simulink library "mach_lib"  (Simulink 6.3)
undefined symbols (not defined in the file): accel_cmd, aero_surf_qbar_off, aero_surf_qbar_on, altitude_stop, angular_rate_stop, att_cmd_select, att_trim_IC, att_type, att_type_numbers, bb_ellipsoid, bb_params, chi_trim_IC, command_time, compute_all_rate_cols, compute_all_vel_cols, constants, cosA, da_trim_IC, de_trim_IC, DiscIntNeverNeededParam, dr_trim_IC, dtsim, E_rwy, E_trim_IC, Ed_cmd, Ed_trim_IC, energy_stop, eow_boundary, full_surf_llim, full_surf_ulim, gain_var_struct, gam_cmd_descent, gam_cmd_preflare, gamdot_cmd_descent, gamdot_cmd_flare, gamdot_cmd_preflare, gamma_trim_IC, h_trim_IC, hd_cmd, hd_trim_IC, ideal_vel_Kb, integrate_start_time_sim, integrate_state_sim, llim, MACH, MACH_att_fb, MACH_gain_mat, MACH_mass_IC, MACH_pos_IC, MACH_pqr_Bmat_IC, MACH_pqr_IC, MACH_pqr_u_IC, MACH_quat_IC, MACH_throttle_IC, MACH_U_nom_IC, MACH_vel_Bmat_IC, MACH_vel_cvdnom_IC, MACH_vel_IC, MACH_vel_uold_IC, max_chi_cmd ... (+67)
libraries: simulink x75, mach_lib x27, utility_lib x25, model_lib x7, models x6
(part 2 of 6)

== system mach_lib/claw_main/pos_loops ==
  signal_bus : Inport
  outer_cmd : Inport  Port=2
  inner_cmd : Inport  Port=3
  Bus Creator : BusCreator  Inputs=5
  Bus Selector : BusSelector  OutputSignals=feed_forward.pos_ff,mode_sw.int_reset_sw,control_params.pos_desdyn,y_meas.dc_fltpath
  Bus Selector1 : BusSelector  OutputSignals=x_est.NEh
  Mux : Mux  Inputs=[3 1 ]
  P+I+AW+TRIM Control : mach_lib/P+I+AW+TRIM Control
  Product : Product  Multiplication=Matrix(*)  RndMeth=Zero
  Selector1 : Selector  Elements=[1 2 4]  InputPortWidth=4
  Selector3 : Selector  Elements=[1 2 4 3]  InputPortWidth=4
  compute trim : Subsystem
  limiter : Subsystem
  select pos cmd : Subsystem
  d_cmd : Outport
  outputs : Outport  Port=2
  cmd : Outport  Port=3
  wires:
  select pos cmd/2(cam_cmd) -> [camcmd]
  Bus Selector/1 -> P+I+AW+TRIM Control/3  "<pos_ff>"
  limiter/2(cvd_extra) -> [cvdex], Bus Creator/1  "cvdex"
  Product/1 -> Bus Creator/5  "cvdex_fltpath"
  Bus Selector/4 -> Product/1  "<dc_fltpath>"
  Bus Creator/1 -> outputs/1
  P+I+AW+TRIM Control/2 -> Bus Creator/2  "integ"
  [cvdex] -> Product/2
  P+I+AW+TRIM Control/1 -> limiter/3(cvd_des_in)
  limiter/1(cvd_des) -> compute trim/2(cmd), Mux/1
  Bus Selector/3 -> P+I+AW+TRIM Control/7  "<pos_desdyn>"
  Bus Selector/2 -> P+I+AW+TRIM Control/6  "<int_reset_sw>"
  [cvdex] -> P+I+AW+TRIM Control/4
  [trim] -> P+I+AW+TRIM Control/5
  [cv] -> Bus Creator/4  "cv"
  [cvc] -> Bus Creator/3  "cvc"
  Selector3/1 -> d_cmd/1
  select pos cmd/3(cmd) -> cmd/1
  outer_cmd/1 -> select pos cmd/2(outer cmd)
  Selector1/1 -> limiter/1(vel_inner_cmd), compute trim/1(inner cmd)
  inner_cmd/1 -> Selector1/1
  compute trim/1(trim) -> [trim]
  signal_bus/1 -> limiter/2(signal_bus), Bus Selector1/1, select pos cmd/3(signal_bus), Bus Selector/1
  Bus Selector1/1 -> select pos cmd/1(NEh_current), [cv], P+I+AW+TRIM Control/1  "<NEh>"
  select pos cmd/1(NEh_cmd) -> [cvc], P+I+AW+TRIM Control/2
  Mux/1 -> Selector3/1
  [camcmd] -> Mux/2

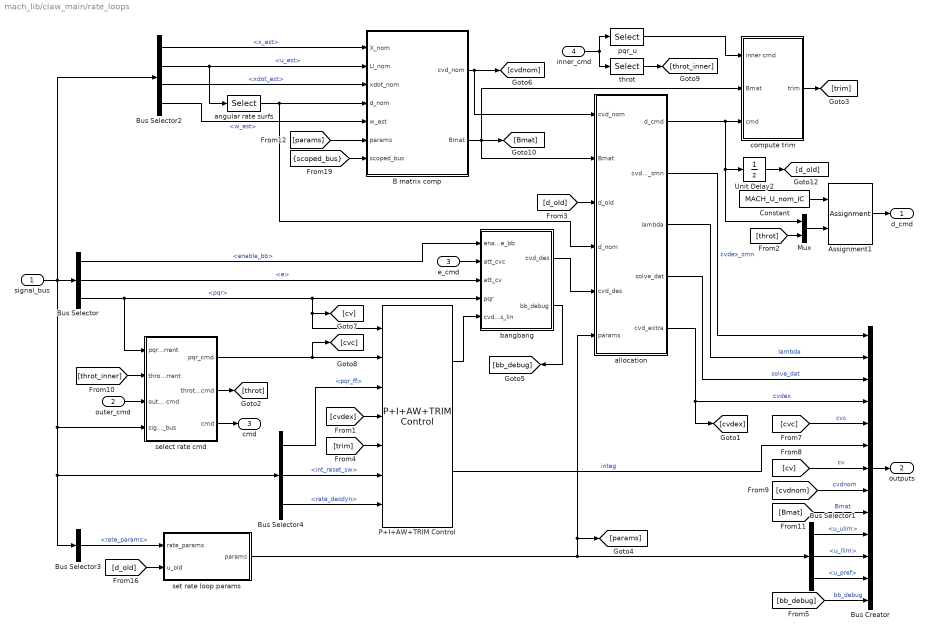
== system mach_lib/claw_main/rate_loops ==
  signal_bus : Inport
  outer_cmd : Inport  Port=2
  e_cmd : Inport  Port=3
  inner_cmd : Inport  Port=4
  Assignment1 : Assignment  Elements=[MACH.pqr_u_idx MACH.throttle_idx]  OutputInitialize=Initialize using input (U1)
  B matrix comp : Subsystem  TreatAsAtomicUnit=on
  Bus Creator : BusCreator  Inputs=13
  Bus Selector : BusSelector  OutputSignals=control_params.enable_bb,x_est.e,x_est.pqr
  Bus Selector1 : BusSelector  OutputSignals=u_ulim,u_llim,u_pref
  Bus Selector2 : BusSelector  OutputSignals=x_est,u_est,xdot_est,y_meas.w_est
  Bus Selector3 : BusSelector  OutputSignals=control_params.rate_params
  Bus Selector4 : BusSelector  OutputSignals=feed_forward.pqr_ff,mode_sw.int_reset_sw,control_params.rate_desdyn
  Constant : Constant  Value=MACH_U_nom_IC
  Mux : Mux  Inputs=2
  P+I+AW+TRIM Control : mach_lib/P+I+AW+TRIM Control
  Unit Delay2 : UnitDelay  X0=MACH_pqr_u_IC  SampleTime=-1
  allocation : Subsystem
  angular rate surfs : Selector  Elements=MACH.pqr_u_idx  InputPortWidth=MACH.num_u
  bangbang : Subsystem
  compute trim : Subsystem
  pqr_u : Selector  Elements=MACH.pqr_u_idx  InputPortWidth=MACH.num_u
  select rate cmd : Subsystem
  set rate loop params : Subsystem
  throt : Selector  Elements=MACH.throttle_idx  InputPortWidth=MACH.num_u
  d_cmd : Outport
  outputs : Outport  Port=2
  cmd : Outport  Port=3
  wires:
  Bus Selector3/1 -> set rate loop params/1(rate_params)  "<rate_params>"
  select rate cmd/3(cmd) -> cmd/1
  [bb_debug] -> Bus Creator/13  "bb_debug"
  bangbang/2(bb_debug) -> [bb_debug]
  Bus Selector/1 -> bangbang/1(enable_bb)  "<enable_bb>"
  P+I+AW+TRIM Control/1 -> bangbang/5(cvd_des_lin)
  Bus Selector/2 -> bangbang/3(att_cv)  "<e>"
  e_cmd/1 -> bangbang/2(att_cvc)
  bangbang/1(cvd_des) -> allocation/5(cvd_des)
  allocation/2(cvd_extra_smn) -> Bus Creator/1  "cvdex_smn"
  Bus Selector4/3 -> P+I+AW+TRIM Control/7  "<rate_desdyn>"
  [params] -> B matrix comp/6(params)
  [scoped_bus] -> B matrix comp/7(scoped_bus)
  Bus Creator/1 -> outputs/1
  allocation/4(solve_dat) -> Bus Creator/3  "solve_dat"
  allocation/3(lambda) -> Bus Creator/2  "lambda"
  B matrix comp/2(Bmat) -> allocation/2(Bmat), [Bmat], compute trim/2(Bmat)
  [d_old] -> allocation/3(d_old)
  allocation/1(d_cmd) -> Unit Delay2/1, Mux/1, compute trim/3(cmd)
  Unit Delay2/1 -> [d_old]
  [throt] -> Mux/2
  allocation/5(cvd_extra) -> [cvdex], Bus Creator/4  "cvdex"
  Bus Selector1/3 -> Bus Creator/12  "<u_pref>"
  Bus Selector2/4 -> B matrix comp/5(w_est)  "<w_est>"
  Bus Selector2/3 -> B matrix comp/3(xdot_nom)  "<xdot_est>"
  Bus Selector2/2 -> B matrix comp/2(U_nom), angular rate surfs/1  "<u_est>"
  Bus Selector2/1 -> B matrix comp/1(X_nom)  "<x_est>"
  Mux/1 -> Assignment1/2
  Constant/1 -> Assignment1/1
  pqr_u/1 -> compute trim/1(inner cmd)
  [d_old] -> set rate loop params/2(u_old)
  Bus Selector1/2 -> Bus Creator/11  "<u_llim>"
  Bus Selector1/1 -> Bus Creator/10  "<u_ulim>"
  [Bmat] -> Bus Creator/9  "Bmat"
  Bus Selector4/2 -> P+I+AW+TRIM Control/6  "<int_reset_sw>"
  Bus Selector4/1 -> P+I+AW+TRIM Control/3  "<pqr_ff>"
  Bus Selector/3 -> [cv], P+I+AW+TRIM Control/1, bangbang/4(pqr), select rate cmd/1(pqr_current)  "<pqr>"
  [cvdex] -> P+I+AW+TRIM Control/4
  [trim] -> P+I+AW+TRIM Control/5
  throt/1 -> [throt_inner]
  Assignment1/1 -> d_cmd/1
  set rate loop params/1(params) -> [params], allocation/6(params), Bus Selector1/1
  [cvdnom] -> Bus Creator/8  "cvdnom"
  [cv] -> Bus Creator/7  "cv"
  [cvc] -> Bus Creator/5  "cvc"
  [throt_inner] -> select rate cmd/2(throt_current)
  select rate cmd/1(pqr_cmd) -> P+I+AW+TRIM Control/2, [cvc]
  select rate cmd/2(throt_cmd) -> [throt]
  inner_cmd/1 -> throt/1, pqr_u/1
  compute trim/1(trim) -> [trim]
  signal_bus/1 -> select rate cmd/4(signal_bus), Bus Selector4/1, Bus Selector3/1, Bus Selector/1, Bus Selector2/1
  P+I+AW+TRIM Control/2 -> Bus Creator/6  "integ"
  B matrix comp/1(cvd_nom) -> allocation/1(cvd_nom), [cvdnom]
  outer_cmd/1 -> select rate cmd/3(outer cmd)
  angular rate surfs/1 -> allocation/4(d_nom), B matrix comp/4(d_nom)

== system mach_lib/claw_main/servo commands  when not engaged ==
  note: for OAV/MAV during "pre-takeoff",
      |  the rate inner_cmd throt was set to takeoff throt
      | to allow integrators to trim for anticipated takeoff.
      | This should be revisited within current CLAW
      | before being used again.
  signal_bus : Inport
  outer_cmd : Inport  Port=2
  Bus Selector1 : BusSelector  OutputSignals=mode_sw.pre_takeoff_sw,mode_sw.engaged_sw,mode_sw.full_surf_cmd_sw,cmd_bus.autopilot_cmd,full_surf.full_surf_cmd
  Constant1 : Constant  Value=MACH.pre_takeoff_u_backtrim
  Multiport Switch : MultiPortSwitch  Inputs=2  zeroidx=on
  Multiport Switch1 : MultiPortSwitch  Inputs=2  zeroidx=on
  Multiport Switch2 : MultiPortSwitch  Inputs=2  zeroidx=on
  pseudo surf cmd : Subsystem
  u_out : Outport
  u_backtrim : Outport  Port=2
  wires:
  Multiport Switch/1 -> u_backtrim/1
  outer_cmd/1 -> Multiport Switch1/3
  Multiport Switch2/1 -> Multiport Switch1/2
  Bus Selector1/5 -> Multiport Switch2/3  "<full_surf_cmd>"
  pseudo surf cmd/1(surf_cmd) -> Multiport Switch2/2
  Bus Selector1/4 -> pseudo surf cmd/1(autopilot_cmd)  "<autopilot_cmd>"
  Bus Selector1/3 -> Multiport Switch2/1  "<full_surf_cmd_sw>"
  Bus Selector1/2 -> Multiport Switch1/1  "<engaged_sw>"
  Constant1/1 -> Multiport Switch/3
  Multiport Switch1/1 -> u_out/1, Multiport Switch/2
  Bus Selector1/1 -> Multiport Switch/1  "<pre_takeoff_sw>"
  signal_bus/1 -> Bus Selector1/1

== system mach_lib/claw_main/set scoped signals ==
  signal_bus : Inport
  Bus Selector3 : BusSelector  OutputSignals=y_meas.h_geodetic,mode_sw.use_held_aero_obac_sw,y_meas.w_est,y_meas.NEh_dot,mode_sw.att_type,u_est,engines
  Gain1 : Gain  Orientation=left  Gain=use_variable_mass
  hold altitude : model_lib/hold input
  mass : DiscreteIntegrator  gainval=1  InitialCondition=MACH_mass_IC  SampleTime=-1  ICPrevOutput=DiscIntNeverNeededParam  ICPrevScaledInput=DiscIntNeverNeededParam
  set scoped bus : model_lib/set scoped bus  vehicle_params=obac_params
  set scoped signals : model_lib/set scoped signals
  scoped_bus : Outport
  wires:
  Bus Selector3/7 -> set scoped bus/6  "<engines>"
  Bus Selector3/6 -> set scoped bus/5  "<u_est>"
  Bus Selector3/5 -> set scoped bus/4  "<att_type>"
  Bus Selector3/4 -> set scoped bus/3  "<NEh_dot>"
  Bus Selector3/3 -> set scoped bus/2  "<w_est>"
  hold altitude/1 -> set scoped bus/1
  Bus Selector3/2 -> hold altitude/2  "<use_held_aero_obac_sw>"
  mass/1 -> set scoped bus/7
  set scoped bus/1 -> scoped_bus/1, set scoped signals/1
  set scoped bus/2 -> Gain1/1
  Bus Selector3/1 -> hold altitude/1  "<h_geodetic>"
  Gain1/1 -> mass/1
  signal_bus/1 -> Bus Selector3/1

== system mach_lib/claw_main/state est ==
  u_old : Inport
  sensors : Inport  Port=2
  signal_bus : Inport  Port=3
  Bus Creator : BusCreator  Inputs=12
  Bus Creator1 : BusCreator  Inputs=6
  Bus Selector : BusSelector  OutputSignals=mode_sw.reset_pos_sw,mode_sw.nav_enable_sw,mode_sw.wind_est_sw
  Bus Selector1 : BusSelector  OutputSignals=nav_ok,pqr,NED_dot,latlonh,e
  Bus Selector2 : BusSelector  OutputSignals=aero_env.Mach,aero_env.vel,aero_env.alpha,aero_env.beta,aero_env.uvw_rw,aero_env.qbar
  Bus Selector3 : BusSelector  OutputSignals=u_meas,seeker,accels_cg
  Logical Operator : Logic  AllPortsSameDT=off  OutDataTypeMode=Boolean
  beta_360 : Fcn  Expr=atan2(u(2),u(1))
  cl model : models/datcom-obac
  process inputs : Subsystem
  process sensors : Subsystem
  wind estimator : Subsystem
  y_meas : Outport
  x_est : Outport  Port=2
  xdot_est : Outport  Port=3
  u_est : Outport  Port=4
  aero_env_est : Outport  Port=5
  w_est_debug : Outport  Port=6
  wires:
  Bus Creator/1 -> y_meas/1
  Bus Selector3/3 -> Bus Creator/3  "<accels_cg>"
  Bus Selector3/2 -> Bus Creator/2  "<seeker>"
  Bus Selector3/1 -> Bus Creator/1  "<u_meas>"
  Bus Selector2/6 -> Bus Creator1/6  "<qbar>"
  Bus Selector2/4 -> Bus Creator1/4  "<beta>"
  Bus Selector2/3 -> Bus Creator1/3  "<alpha>"
  Bus Selector2/2 -> Bus Creator1/2  "<vel>"
  Bus Selector2/1 -> Bus Creator1/1  "<Mach>"
  beta_360/1 -> Bus Creator1/5  "beta_360"
  process sensors/6(dc_fltpath) -> Bus Creator/9  "dc_fltpath"
  Bus Selector2/5 -> beta_360/1  "<uvw_rw>"
  Bus Selector/2 -> Logical Operator/1  "<nav_enable_sw>"
  Bus Selector1/1 -> Logical Operator/2  "<nav_ok>"
  Logical Operator/1 -> process sensors/2(nav_ok)
  Bus Creator1/1 -> aero_env_est/1
  cl model/2 -> Bus Selector2/1
  wind estimator/2(w_est_debug) -> w_est_debug/1
  u_old/1 -> process inputs/1(u_old)
  process sensors/7(cvc_origin) -> Bus Creator/10  "cvc_origin"
  process sensors/1(vehicle_origin) -> Bus Creator/4  "vehicle_origin"
  process sensors/5(NEh_dot) -> Bus Creator/8  "NEh_dot"
  process sensors/4(nav_valid) -> Bus Creator/7  "nav_valid"
  process sensors/3(NEh_nav) -> Bus Creator/6  "NEh_nav"
  process sensors/2(h_geodetic) -> Bus Creator/5  "h_geodetic"
  Bus Selector1/5 -> process sensors/6(e)  "<e>"
  Bus Selector1/4 -> process sensors/5(latlonh)  "<latlonh>"
  Bus Selector1/3 -> process sensors/4(NED_dot)  "<NED_dot>"
  Bus Selector1/2 -> process sensors/3(pqr)  "<pqr>"
  process inputs/1(u_est) -> wind estimator/4(u), cl model/2, u_est/1
  Bus Selector/3 -> wind estimator/5(wind_est_sw)  "<wind_est_sw>"
  Bus Selector/1 -> process sensors/1(reset_pos)  "<reset_pos_sw>"
  signal_bus/1 -> Bus Selector/1
  process sensors/9(x_est) -> x_est/1, wind estimator/2(x), cl model/1
  cl model/1 -> xdot_est/1
  process sensors/8(dircos) -> Bus Creator/11, wind estimator/1(dircos)  "dircos"
  wind estimator/1(w_est) -> Bus Creator/12, cl model/3  "w_est"
  sensors/1 -> Bus Selector1/1, wind estimator/3(sensors), process inputs/2(sensors), Bus Selector3/1

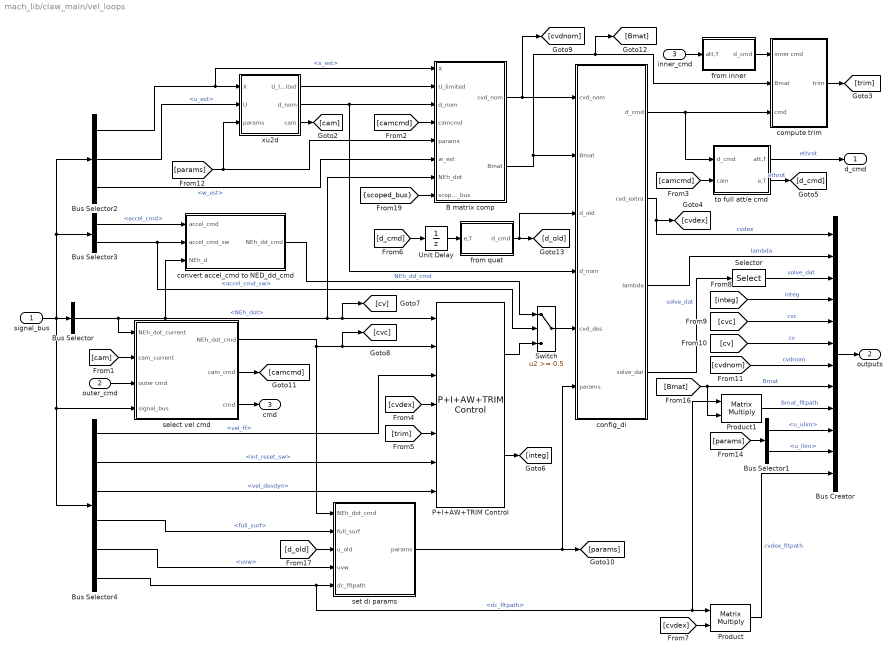
== system mach_lib/claw_main/vel_loops ==
  signal_bus : Inport
  outer_cmd : Inport  Port=2
  inner_cmd : Inport  Port=3
  B matrix comp : Subsystem
  Bus Creator : BusCreator  Inputs=12
  Bus Selector : BusSelector  OutputSignals=y_meas.NEh_dot
  Bus Selector1 : BusSelector  OutputSignals=u_ulim,u_llim
  Bus Selector2 : BusSelector  OutputSignals=x_est,u_est,y_meas.w_est
  Bus Selector3 : BusSelector  OutputSignals=control_params.accel_cmd,control_params.accel_cmd_sw
  Bus Selector4 : BusSelector  OutputSignals=feed_forward.vel_ff,mode_sw.int_reset_sw,control_params.vel_desdyn,full_surf,x_est.uvw,y_meas.dc_fltpath
  P+I+AW+TRIM Control : mach_lib/P+I+AW+TRIM Control
  Product : Product  Multiplication=Matrix(*)  RndMeth=Zero
  Product1 : Product  Multiplication=Matrix(*)  RndMeth=Zero
  Selector : Selector  InputType=Matrix  Elements=MACH.pqr_u_idx  Rows=1:9  Columns=1:2  InputPortWidth=MACH.num_u
  Switch : Switch  Threshold=0.5
  Unit Delay : UnitDelay  X0=MACH_vel_uold_IC  SampleTime=-1
  compute trim : Subsystem
  config_di : Subsystem  BlockChoice=di_smn  mask{num_cv=MACH.vel_num_cv, num_u=MACH.vel_num_u, wght_cv_type=MACH.vel_wght_cv_type}
      link override di_smn/config_smn/smn_sfunc: sfunc_name=MACH.smn_sfunc_name
      link override di_smn/config_smn/smn_sfunc/S-Function: FunctionName=smn_sfunc_gam_mpass_epsposdef
      settings: AttributesFormatString=%<BlockChoice>  TemplateBlock=mach_lib/config_di  MemberBlocks=di_pseudoinv,di_smn
  convert accel_cmd to NED_dd_cmd : Subsystem  TreatAsAtomicUnit=on
  from inner : Subsystem
  from quat : Subsystem
  select vel cmd : Subsystem
  set di params : Subsystem
  to full att/e cmd : Subsystem
  xu2d : Subsystem
  d_cmd : Outport
  outputs : Outport  Port=2
  cmd : Outport  Port=3
  wires:
  Bus Creator/1 -> outputs/1
  select vel cmd/1(NEh_dot_cmd) -> [cvc], P+I+AW+TRIM Control/2, set di params/1(NEh_dot_cmd)
  select vel cmd/2(cam_cmd) -> [camcmd]
  select vel cmd/3(cmd) -> cmd/1
  outer_cmd/1 -> select vel cmd/3(outer cmd)
  to full att/e cmd/2(e,T) -> [d_cmd]  "ethrot"
  Bus Selector4/6 -> set di params/5(dc_fltpath), Product1/1, Product/1  "<dc_fltpath>"
  Product1/1 -> Bus Creator/9  "Bmat_fltpath"
  Bus Selector3/2 -> Switch/2, convert accel_cmd to NED_dd_cmd/2(accel_cmd_sw)  "<accel_cmd_sw>"
  signal_bus/1 -> select vel cmd/4(signal_bus), Bus Selector4/1, Bus Selector2/1, Bus Selector3/1, Bus Selector/1
  convert accel_cmd to NED_dd_cmd/1(NEh_dd_cmd) -> Switch/1  "NEh_dd_cmd"
  P+I+AW+TRIM Control/1 -> Switch/3
  Switch/1 -> config_di/5(cvd_des)
  Bus Selector3/1 -> convert accel_cmd to NED_dd_cmd/1(accel_cmd)  "<accel_cmd>"
  Bus Selector4/3 -> P+I+AW+TRIM Control/7  "<vel_desdyn>"
  Bus Selector2/2 -> xu2d/2(U)  "<u_est>"
  Bus Selector2/1 -> B matrix comp/1(X), xu2d/1(X)  "<x_est>"
  [scoped_bus] -> B matrix comp/8(scoped_bus)
  [camcmd] -> B matrix comp/4(camcmd)
  Selector/1 -> Bus Creator/3  "solve_dat"
  [cvdex] -> Product/2
  config_di/4(solve_dat) -> Selector/1  "solve_dat"
  config_di/3(lambda) -> Bus Creator/2  "lambda"
  Bus Selector4/5 -> set di params/4(uvw)  "<uvw>"
  [d_old] -> set di params/3(u_old)
  Bus Selector1/2 -> Bus Creator/11  "<u_llim>"
  Bus Selector1/1 -> Bus Creator/10  "<u_ulim>"
  [params] -> Bus Selector1/1
  Product/1 -> Bus Creator/12  "cvdex_fltpath"
  Bus Selector4/4 -> set di params/2(full_surf)  "<full_surf>"
  from quat/1(d_cmd) -> config_di/3(d_old), [d_old]
  config_di/2(cvd_extra) -> Bus Creator/1, [cvdex]  "cvdex"
  [Bmat] -> Bus Creator/8, Product1/2  "Bmat"
  B matrix comp/1(cvd_nom) -> config_di/1(cvd_nom), [cvdnom]
  Bus Selector4/1 -> P+I+AW+TRIM Control/3  "<vel_ff>"
  Bus Selector4/2 -> P+I+AW+TRIM Control/6  "<int_reset_sw>"
  [cvdex] -> P+I+AW+TRIM Control/4
  [trim] -> P+I+AW+TRIM Control/5
  [cvdnom] -> Bus Creator/7  "cvdnom"
  [cv] -> Bus Creator/6  "cv"
  [cvc] -> Bus Creator/5  "cvc"
  [integ] -> Bus Creator/4  "integ"
  xu2d/1(U_limited) -> B matrix comp/2(U_limited)
  [params] -> B matrix comp/5(params), xu2d/3(params)
  set di params/1(params) -> config_di/6(params), [params]
  Unit Delay/1 -> from quat/1(e,T)
  [d_cmd] -> Unit Delay/1
  Bus Selector2/3 -> B matrix comp/6(w_est)  "<w_est>"
  [camcmd] -> to full att/e cmd/2(cam)
  from inner/1(d_cmd) -> compute trim/1(inner cmd)
  inner_cmd/1 -> from inner/1(att,T)
  compute trim/1(trim) -> [trim]
  [cam] -> select vel cmd/2(cam_current)
  xu2d/3(cam) -> [cam]
  Bus Selector/1 -> select vel cmd/1(NEh_dot_current), [cv], P+I+AW+TRIM Control/1, B matrix comp/7(NEh_dot), convert accel_cmd to NED_dd_cmd/3(NEh_d)  "<NEh_dot>"
  xu2d/2(d_nom) -> B matrix comp/3(d_nom), config_di/4(d_nom)
  P+I+AW+TRIM Control/2 -> [integ]
  config_di/1(d_cmd) -> to full att/e cmd/1(d_cmd), compute trim/3(cmd)
  to full att/e cmd/1(att,T) -> d_cmd/1  "ethrot"
  B matrix comp/2(Bmat) -> [Bmat], compute trim/2(Bmat), config_di/2(Bmat)

== system mach_lib/control input/form control input ==
  cmd_bus : Inport
  Bus Creator : BusCreator
  Bus Selector4 : BusSelector  OutputSignals=command,full_surf_cmd
  add effector control params : Subsystem
  engine parameters : Subsystem
  mode switches : Subsystem
  select command : Subsystem
  control_input : Outport
  wires:
  Bus Creator/1 -> control_input/1
  cmd_bus/1 -> select command/1(cmd_bus)
  mode switches/1(mode_sw) -> Bus Creator/3  "mode_sw"
  engine parameters/1(engines) -> Bus Creator/4  "engines"
  Bus Selector4/2 -> add effector control params/1(full_surf_cmd)  "<full_surf_cmd>"
  add effector control params/1(full_surf) -> Bus Creator/2  "full_surf"
  Bus Selector4/1 -> Bus Creator/1  "<command>"
  select command/1(control_input) -> mode switches/1(control_input), Bus Selector4/1

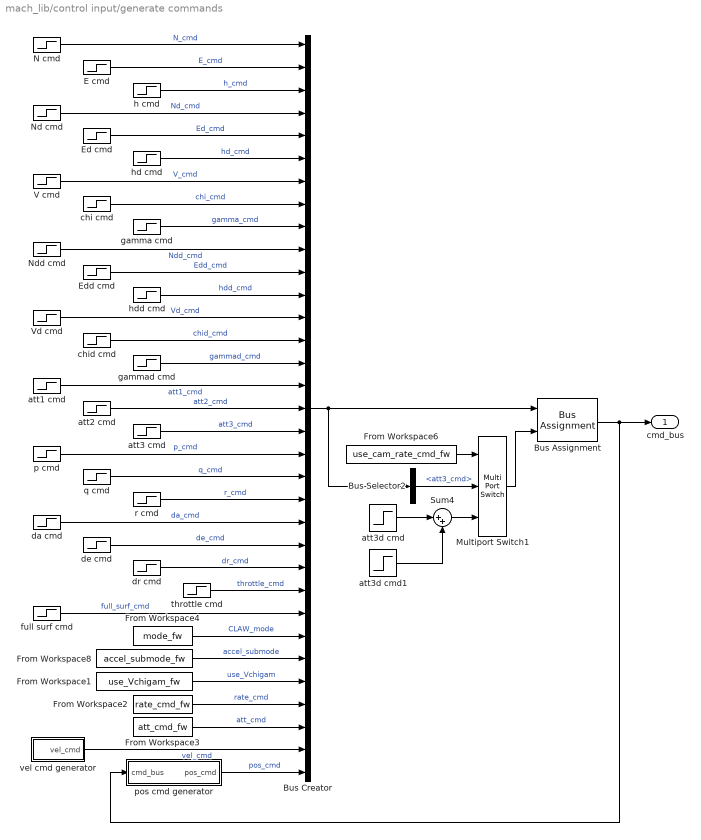
== system mach_lib/control input/generate commands ==
  Bus Assignment : BusAssignment  AssignedSignals=att3_cmd
  Bus Creator : BusCreator  Inputs=33
  Bus Selector2 : BusSelector  OutputSignals=att3_cmd
  E cmd : Step  Time=command_time  Before=E_trim_IC  After=E_trim_IC+10*0  SampleTime=MACH.dt
  Ed cmd : Step  Time=command_time  Before=Ed_trim_IC  After=Ed_trim_IC  SampleTime=MACH.dt
  Edd cmd : Step  Time=command_time  After=0  SampleTime=MACH.dt
  From Workspace1 : FromWorkspace  VariableName=use_Vchigam_fw  SampleTime=MACH.dt  Interpolate=off  OutputAfterFinalValue=Holding final value
  From Workspace2 : FromWorkspace  VariableName=rate_cmd_fw  SampleTime=MACH.dt  OutputAfterFinalValue=Holding final value
  From Workspace3 : FromWorkspace  VariableName=att_cmd_fw  SampleTime=MACH.dt  OutputAfterFinalValue=Holding final value
  From Workspace4 : FromWorkspace  VariableName=mode_fw  SampleTime=MACH.dt  Interpolate=off  OutputAfterFinalValue=Holding final value
  From Workspace6 : FromWorkspace  VariableName=use_cam_rate_cmd_fw  SampleTime=MACH.dt  Interpolate=off  OutputAfterFinalValue=Holding final value
  From Workspace8 : FromWorkspace  VariableName=accel_submode_fw  SampleTime=MACH.dt  Interpolate=off  OutputAfterFinalValue=Holding final value
  Multiport Switch1 : MultiPortSwitch  Inputs=2  zeroidx=on
  N cmd : Step  Time=command_time  Before=N_trim_IC  After=N_trim_IC+10*0  SampleTime=MACH.dt
  Nd cmd : Step  Time=command_time  Before=Nd_trim_IC  After=Nd_trim_IC  SampleTime=MACH.dt
  Ndd cmd : Step  Time=command_time  After=0  SampleTime=MACH.dt
  Sum4 : Sum  Inputs=|++  SaturateOnIntegerOverflow=on
  V cmd : Step  Time=command_time  Before=V_trim_IC  After=V_trim_IC  SampleTime=MACH.dt
  Vd cmd : Step  Time=command_time  After=0  SampleTime=MACH.dt
  att1 cmd : Step  Tag=tilta  Time=command_time  Before=att_trim_IC(1)  After=att_trim_IC(1) + 0.1*0  SampleTime=MACH.dt
      settings: AttributesFormatString=%<Name> (%<Tag>)
  att2 cmd : Step  Tag=tiltb  Description=theta  Time=command_time  Before=att_trim_IC(2)  After="att_trim_IC(2)  + 0.1*0"  SampleTime=MACH.dt
      settings: AttributesFormatString=%<Name> (%<Tag>)
  att3 cmd : Step  Tag=cam  Time=command_time  Before=att_trim_IC(3)  After="att_trim_IC(3)  + 0.1*0"  SampleTime=MACH.dt
      settings: AttributesFormatString=%<Name> (%<Tag>)
  att3d cmd : Step  Tag=cam  Time=command_time + (15 - command_time)  After=-0.04*0  SampleTime=MACH.dt
      settings: AttributesFormatString=%<Name> (%<Tag>)
  att3d cmd1 : Step  Time=command_time + (17 - command_time)  After=0.04*0  SampleTime=MACH.dt
  chi cmd : Step  Time=command_time  Before=chi_trim_IC  After=chi_trim_IC  SampleTime=MACH.dt
  chid cmd : Step  Time=command_time  After=0  SampleTime=MACH.dt
  da cmd : Step  Time=command_time  Before=da_trim_IC  After=da_trim_IC  SampleTime=MACH.dt
  de cmd : Step  Time=command_time  Before=de_trim_IC  After=de_trim_IC  SampleTime=MACH.dt
  dr cmd : Step  Time=command_time  Before=dr_trim_IC  After=dr_trim_IC  SampleTime=MACH.dt
  full surf cmd : Step  Time=command_time  Before=MACH_U_nom_IC  After=MACH_U_nom_IC  SampleTime=MACH.dt
  gamma cmd : Step  Time=command_time  Before=gamma_trim_IC  After=gamma_trim_IC  SampleTime=MACH.dt
  gammad cmd : Step  Time=command_time  After=0  SampleTime=MACH.dt
  h cmd : Step  Time=command_time  Before=h_trim_IC  After=h_trim_IC + 10*0  SampleTime=MACH.dt
  hd cmd : Step  Time=command_time  Before=hd_trim_IC  After=hd_trim_IC  SampleTime=MACH.dt
  hdd cmd : Step  Time=command_time  After=0  SampleTime=MACH.dt
  p cmd : Step  Time=command_time  Before=pqr_trim_IC(1)  After=pqr_trim_IC(1) + 0.2*0  SampleTime=MACH.dt
  pos cmd generator : Subsystem
  q cmd : Step  Time=command_time  Before=pqr_trim_IC(2)  After=pqr_trim_IC(2) + 0.2*0  SampleTime=MACH.dt
  r cmd : Step  Time=command_time  Before=pqr_trim_IC(3)  After=pqr_trim_IC(3) + 0.2*0  SampleTime=MACH.dt
  throttle cmd : Step  Time=command_time  Before=throttle_trim_IC(1)  After=throttle_trim_IC(1)  SampleTime=MACH.dt
  vel cmd generator : Subsystem
  cmd_bus : Outport
  wires:
  Bus Creator/1 -> Bus Assignment/1, Bus Selector2/1
  throttle cmd/1 -> Bus Creator/25  "throttle_cmd"
  dr cmd/1 -> Bus Creator/24  "dr_cmd"
  de cmd/1 -> Bus Creator/23  "de_cmd"
  da cmd/1 -> Bus Creator/22  "da_cmd"
  r cmd/1 -> Bus Creator/21  "r_cmd"
  q cmd/1 -> Bus Creator/20  "q_cmd"
  p cmd/1 -> Bus Creator/19  "p_cmd"
  att3 cmd/1 -> Bus Creator/18  "att3_cmd"
  att2 cmd/1 -> Bus Creator/17  "att2_cmd"
  att1 cmd/1 -> Bus Creator/16  "att1_cmd"
  hd cmd/1 -> Bus Creator/6  "hd_cmd"
  Ed cmd/1 -> Bus Creator/5  "Ed_cmd"
  Nd cmd/1 -> Bus Creator/4  "Nd_cmd"
  h cmd/1 -> Bus Creator/3  "h_cmd"
  E cmd/1 -> Bus Creator/2  "E_cmd"
  N cmd/1 -> Bus Creator/1  "N_cmd"
  From Workspace6/1 -> Multiport Switch1/1
  Sum4/1 -> Multiport Switch1/3
  att3d cmd/1 -> Sum4/1
  att3d cmd1/1 -> Sum4/2
  Bus Selector2/1 -> Multiport Switch1/2  "<att3_cmd>"
  Multiport Switch1/1 -> Bus Assignment/2
  Bus Assignment/1 -> pos cmd generator/1(cmd_bus), cmd_bus/1
  From Workspace3/1 -> Bus Creator/31  "att_cmd"
  vel cmd generator/1(vel_cmd) -> Bus Creator/32  "vel_cmd"
  pos cmd generator/1(pos_cmd) -> Bus Creator/33  "pos_cmd"
  From Workspace4/1 -> Bus Creator/27  "CLAW_mode"
  From Workspace8/1 -> Bus Creator/28  "accel_submode"
  full surf cmd/1 -> Bus Creator/26  "full_surf_cmd"
  Ndd cmd/1 -> Bus Creator/10  "Ndd_cmd"
  Edd cmd/1 -> Bus Creator/11  "Edd_cmd"
  hdd cmd/1 -> Bus Creator/12  "hdd_cmd"
  Vd cmd/1 -> Bus Creator/13  "Vd_cmd"
  chid cmd/1 -> Bus Creator/14  "chid_cmd"
  gammad cmd/1 -> Bus Creator/15  "gammad_cmd"
  V cmd/1 -> Bus Creator/7  "V_cmd"
  chi cmd/1 -> Bus Creator/8  "chi_cmd"
  gamma cmd/1 -> Bus Creator/9  "gamma_cmd"
  From Workspace1/1 -> Bus Creator/29  "use_Vchigam"
  From Workspace2/1 -> Bus Creator/30  "rate_cmd"

== system mach_lib/di_pseudoinv/pseudoinv ==
  rhs : Inport
  Bmat : Inport  Port=2
  Math Function : Math  Operator=transpose  SaturateOnIntegerOverflow=on
  Product : Product  Inputs=*/*  Multiplication=Matrix(*)  SaturateOnIntegerOverflow=on  InputSameDT=on
  Product1 : Product  Inputs=**  Multiplication=Matrix(*)  SaturateOnIntegerOverflow=on  InputSameDT=on
  sol : Outport
  wires:
  rhs/1 -> Product/3
  Product/1 -> sol/1
  Product1/1 -> Product/2
  Math Function/1 -> Product/1, Product1/2
  Bmat/1 -> Product1/1, Math Function/1

== system mach_lib/di_smn/config_smn ==
  rhs : Inport
  Bmat : Inport  Port=2
  ulim : Inport  Port=3
  llim : Inport  Port=4
  w_rhs : Inport  Port=5
  sol_pref : Inport  Port=6
  w_pref : Inport  Port=7
  lambda_p : Inport  Port=8
  smn_sfunc : mach_lib/smn_sfunc  sfunc_name=smn_sfunc_name
  sol : Outport
  lambda : Outport  Port=2
  solve_dat : Outport  Port=3
  wires:
  rhs/1 -> smn_sfunc/1
  Bmat/1 -> smn_sfunc/2
  ulim/1 -> smn_sfunc/3
  llim/1 -> smn_sfunc/4
  w_rhs/1 -> smn_sfunc/5
  sol_pref/1 -> smn_sfunc/6
  w_pref/1 -> smn_sfunc/7
  lambda_p/1 -> smn_sfunc/8
  smn_sfunc/1 -> sol/1
  smn_sfunc/2 -> lambda/1
  smn_sfunc/3 -> solve_dat/1

== system mach_lib/di_smn/config_wght_cv ==
  rhs : Inport
  Bmat : Inport  Port=2
  wght_cv : Inport  Port=3
  wght_cv_diag : mach_lib/wght_cv_diag
  rhs_smn : Outport
  Bmat_smn : Outport  Port=2
  wght_cv_smn : Outport  Port=3
  wires:
  rhs/1 -> wght_cv_diag/1
  Bmat/1 -> wght_cv_diag/2
  wght_cv/1 -> wght_cv_diag/3
  wght_cv_diag/1 -> rhs_smn/1
  wght_cv_diag/2 -> Bmat_smn/1
  wght_cv_diag/3 -> wght_cv_smn/1

== system mach_lib/sim params/effector limits ==
  Bus Creator1 : BusCreator  Inputs=6
  From Workspace : FromWorkspace  VariableName=full_surf_limits_fw.trac.llim  SampleTime=dtsim  Interpolate=off  OutputAfterFinalValue=Holding final value
  From Workspace1 : FromWorkspace  VariableName=full_surf_limits_fw.trac.ulim  SampleTime=dtsim  Interpolate=off  OutputAfterFinalValue=Holding final value
  From Workspace3 : FromWorkspace  VariableName=full_surf_limits_fw.trac.lrlim  SampleTime=dtsim  Interpolate=off  OutputAfterFinalValue=Holding final value
  From Workspace4 : FromWorkspace  VariableName=full_surf_limits_fw.trac.urlim  SampleTime=dtsim  Interpolate=off  OutputAfterFinalValue=Holding final value
  From Workspace5 : FromWorkspace  VariableName=full_surf_limits_fw.trac.utlim  SampleTime=dtsim  Interpolate=off  OutputAfterFinalValue=Holding final value
  From Workspace6 : FromWorkspace  VariableName=full_surf_limits_fw.trac.ltlim  SampleTime=dtsim  Interpolate=off  OutputAfterFinalValue=Holding final value
  effector_limits : Outport
  wires:
  From Workspace/1 -> Bus Creator1/2  "u_llim"
  From Workspace1/1 -> Bus Creator1/1  "u_ulim"
  From Workspace4/1 -> Bus Creator1/3  "u_urlim"
  From Workspace3/1 -> Bus Creator1/4  "u_lrlim"
  From Workspace5/1 -> Bus Creator1/5  "u_utlim"
  From Workspace6/1 -> Bus Creator1/6  "u_ltlim"
  Bus Creator1/1 -> effector_limits/1

== system mach_lib/sim params/engines ==
  Bus Creator2 : BusCreator  Inputs=3
  Constant : Constant  Value=trac_params.Isp_sl  SampleTime=dtsim
  Constant1 : Constant  Value=trac_params.Isp_vacuum  SampleTime=dtsim
  Constant2 : Constant  Value=trac_params.throt_to_ff  SampleTime=dtsim
  engines : Outport
  wires:
  Constant2/1 -> Bus Creator2/3  "throt_to_ff"
  Bus Creator2/1 -> engines/1
  Constant1/1 -> Bus Creator2/2  "Isp_vacuum"
  Constant/1 -> Bus Creator2/1  "Isp_sl"

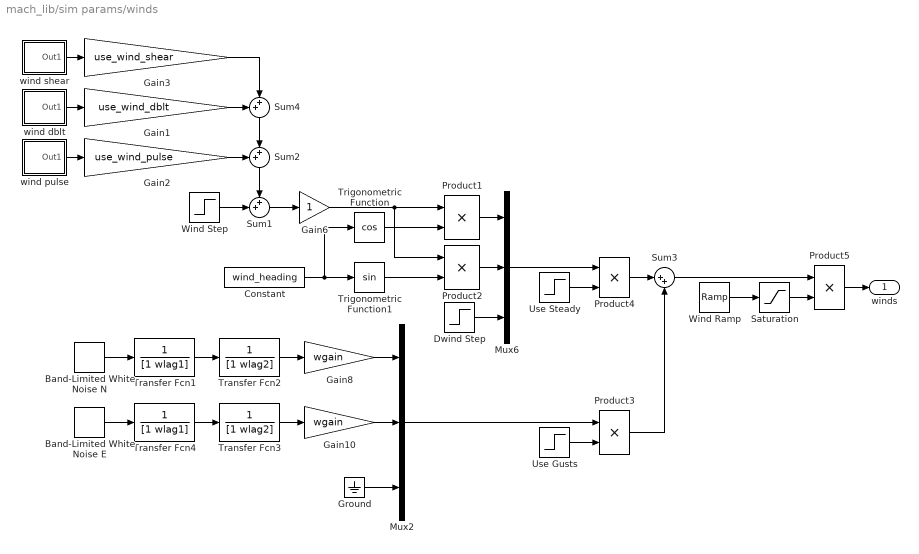
== system mach_lib/sim params/winds ==
  Band-Limited White Noise E : simulink/Sources/Band-Limited White Noise  Cov=1  Ts=dtsim  seed=Eseed
  Band-Limited White Noise N : simulink/Sources/Band-Limited White Noise  Cov=1  Ts=dtsim  seed=Nseed
  Constant : Constant  Value=wind_heading
  Dwind Step : Step  Time=wind_start  After=wind_steady_D  SampleTime=dtsim
  Gain1 : Gain  Gain=use_wind_dblt  SaturateOnIntegerOverflow=on
  Gain10 : Gain  Gain=wgain  SaturateOnIntegerOverflow=on
  Gain2 : Gain  Gain=use_wind_pulse  SaturateOnIntegerOverflow=on
  Gain3 : Gain  Gain=use_wind_shear  SaturateOnIntegerOverflow=on
  Gain6 : Gain  SaturateOnIntegerOverflow=on
  Gain8 : Gain  Gain=wgain  SaturateOnIntegerOverflow=on
  Ground : Ground
  Mux2 : Mux  Inputs=3
  Mux6 : Mux  Inputs=3
  Product1 : Product  SaturateOnIntegerOverflow=on
  Product2 : Product  SaturateOnIntegerOverflow=on
  Product3 : Product  SampleTime=dtsim  SaturateOnIntegerOverflow=on
  Product4 : Product  SampleTime=dtsim  SaturateOnIntegerOverflow=on
  Product5 : Product  SampleTime=dtsim  SaturateOnIntegerOverflow=on
  Saturation : Saturate  UpperLimit=1  LowerLimit=0
  Sum1 : Sum  Inputs=++|  SaturateOnIntegerOverflow=on
  Sum2 : Sum  Orientation=down  Inputs=++|  SaturateOnIntegerOverflow=on
  Sum3 : Sum  Inputs=|++  SaturateOnIntegerOverflow=on
  Sum4 : Sum  Orientation=down  Inputs=++|  SaturateOnIntegerOverflow=on
  Transfer Fcn1 : TransferFcn  Denominator=[1 wlag1]
  Transfer Fcn2 : TransferFcn  Denominator=[1 wlag2]
  Transfer Fcn3 : TransferFcn  Denominator=[1 wlag2]
  Transfer Fcn4 : TransferFcn  Denominator=[1 wlag1]
  Trigonometric Function : Trigonometry  Operator=cos
  Trigonometric Function1 : Trigonometry
  Use Gusts : Step  Time=wind_start  After=use_gusts  SampleTime=dtsim
  Use Steady : Step  Time=wind_start  After=use_steady  SampleTime=dtsim
  Wind Ramp : simulink/Sources/Ramp  slope=wind_slope  start=wind_start  X0=0
  Wind Step : Step  Time=wind_start  After=wind_steady  SampleTime=dtsim
  wind dblt : Subsystem
  wind pulse : Subsystem
  wind shear : Subsystem
  winds : Outport
  wires:
  Saturation/1 -> Product5/2
  Wind Ramp/1 -> Saturation/1
  Sum3/1 -> Product5/1
  Product5/1 -> winds/1
  Sum2/1 -> Sum1/1
  Gain2/1 -> Sum2/1
  Sum4/1 -> Sum2/2
  Gain1/1 -> Sum4/1
  Gain3/1 -> Sum4/2
  wind pulse/1(Out1) -> Gain2/1
  wind dblt/1(Out1) -> Gain1/1
  Gain6/1 -> Product2/1, Product1/1
  Sum1/1 -> Gain6/1
  wind shear/1(Out1) -> Gain3/1
  Mux2/1 -> Product3/1
  Use Steady/1 -> Product4/2
  Use Gusts/1 -> Product3/2
  Gain10/1 -> Mux2/2
  Gain8/1 -> Mux2/1
  Product2/1 -> Mux6/2
  Trigonometric Function1/1 -> Product2/2
  Product1/1 -> Mux6/1
  Trigonometric Function/1 -> Product1/2
  Constant/1 -> Trigonometric Function1/1, Trigonometric Function/1
  Transfer Fcn2/1 -> Gain8/1
  Product3/1 -> Sum3/2
  Ground/1 -> Mux2/3
  Transfer Fcn3/1 -> Gain10/1
  Band-Limited White Noise E/1 -> Transfer Fcn4/1
  Transfer Fcn4/1 -> Transfer Fcn3/1
  Band-Limited White Noise N/1 -> Transfer Fcn1/1
  Transfer Fcn1/1 -> Transfer Fcn2/1
  Product4/1 -> Sum3/1
  Mux6/1 -> Product4/1
  Dwind Step/1 -> Mux6/3
  Wind Step/1 -> Sum1/2

== system mach_lib/claw_main/att_loops/P+I+AW+TRIM Control ==
  cv : Inport
  cv cmd : Inport  Port=2
  cvd ff : Inport  Port=3
  cvdot extra : Inport  Port=4
  trim : Inport  Port=5
  reset : Inport  Port=6
  x0 : Inport  Port=7
  Dot Product2 : simulink/Math Operations/Dot Product  InputSameDT=on  OutDataType=sfix(16)  OutScaling=2^-10  DoSatur=off
  P+I+AW+TRIM Control : mach_lib/P+I+AW+TRIM Control
  Product2 : Product  SaturateOnIntegerOverflow=on  InputSameDT=on
  Sum : Sum  Inputs=-+|  SaturateOnIntegerOverflow=on
  Unit Delay1 : UnitDelay  SampleTime=-1
  fe : Gain  Gain=MACH.att_fe  SaturateOnIntegerOverflow=on
  cvdot des : Outport
  int state : Outport  Port=2
  wires:
  cv/1 -> P+I+AW+TRIM Control/1, Dot Product2/1, Product2/1
  cv cmd/1 -> P+I+AW+TRIM Control/2
  P+I+AW+TRIM Control/1 -> cvdot des/1, Unit Delay1/1
  P+I+AW+TRIM Control/2 -> int state/1
  Dot Product2/1 -> Product2/2
  Unit Delay1/1 -> Dot Product2/2
  Product2/1 -> fe/1
  trim/1 -> Sum/2
  fe/1 -> Sum/1
  x0/1 -> P+I+AW+TRIM Control/7
  reset/1 -> P+I+AW+TRIM Control/6
  Sum/1 -> P+I+AW+TRIM Control/5
  cvdot extra/1 -> P+I+AW+TRIM Control/4
  cvd ff/1 -> P+I+AW+TRIM Control/3

== system mach_lib/claw_main/att_loops/compute trim ==
  inner cmd : Inport
  Bmat : Inport  Port=2
  cmd : Inport  Port=3
  Product : Product  Multiplication=Matrix(*)  SaturateOnIntegerOverflow=on
  Sum1 : Sum  Inputs=|+-  SaturateOnIntegerOverflow=on
  trim : Outport
  wires:
  cmd/1 -> Sum1/2
  inner cmd/1 -> Sum1/1
  Sum1/1 -> Product/2
  Bmat/1 -> Product/1
  Product/1 -> trim/1

== system mach_lib/claw_main/att_loops/dyn inv ==
  limit_pqr_cmd : Inport
  uvw : Inport  Port=2
  e nom : Inport  Port=3
  e dot des : Inport  Port=4
  Dot Product : simulink/Math Operations/Dot Product  InputSameDT=on  OutDataType=sfix(16)  OutScaling=2^-10  DoSatur=off
  Gain4 : Gain  Gain=0.5
  Limit rate cmd : Subsystem
  Product4 : Product  SaturateOnIntegerOverflow=on  InputSameDT=on
  Product5 : Product  Inputs=**  Multiplication=Matrix(*)  SaturateOnIntegerOverflow=on  InputSameDT=on
  Sum4 : Sum  Inputs=++-  SaturateOnIntegerOverflow=on  InputSameDT=on
  getedinv : utility_lib/getedinv
  Bmat : Outport
  pqr : Outport  Port=2
  cvdex : Outport  Port=3
  wires:
  Gain4/1 -> Bmat/1, Product5/1
  limit_pqr_cmd/1 -> Limit rate cmd/1(limit_pqr_cmd)
  getedinv/1 -> Limit rate cmd/3(pqr)
  uvw/1 -> Limit rate cmd/2(uvw)
  getedinv/2 -> Gain4/1
  Dot Product/1 -> Product4/2
  e nom/1 -> getedinv/2, Dot Product/1, Product4/1
  e dot des/1 -> getedinv/1, Sum4/3, Dot Product/2
  Product5/1 -> Sum4/1
  Product4/1 -> Sum4/2
  Sum4/1 -> cvdex/1
  Limit rate cmd/1(pqr_limited) -> Product5/2, pqr/1

== system mach_lib/claw_main/att_loops/low pass filter ==
  e_cmd : Inport
  signal_bus : Inport  Port=2
  att_ff : Inport  Port=3
  Bus Selector4 : BusSelector  OutputSignals=control_params.att_desdyn.kf,control_params.att_desdyn.kb
  Compare To Zero : simulink/Logic and Bit Operations/Compare To Zero  relop===  LogicOutDataTypeMode=boolean  ZeroCross=off
  Constant : Constant  Value=MACH_att_fb
  Discrete-Time Integrator : DiscreteIntegrator  ExternalReset=sampled level  InitialConditionSource=external  SampleTime=-1  ICPrevOutput=DiscIntNeverNeededParam  ICPrevScaledInput=DiscIntNeverNeededParam
  Product : Product  Inputs=3  RndMeth=Zero
  Product1 : Product  RndMeth=Zero
  Product2 : Product  RndMeth=Zero
  Sum : Sum  Inputs=|+-
  Sum1 : Sum  Inputs=++|
  cv cmd : Outport
  cvd ff : Outport  Port=2
  wires:
  Constant/1 -> Product2/1
  Bus Selector4/1 -> Product1/2, Product2/2  "<kf>"
  Product2/1 -> Compare To Zero/1, Product/1
  Bus Selector4/2 -> Product/2  "<kb>"
  Compare To Zero/1 -> Discrete-Time Integrator/2
  Product1/1 -> Sum1/1
  att_ff/1 -> Product1/1
  signal_bus/1 -> Bus Selector4/1
  Discrete-Time Integrator/1 -> cv cmd/1, Sum/2
  Sum1/1 -> cvd ff/1, Discrete-Time Integrator/1
  Sum/1 -> Product/3
  e_cmd/1 -> Discrete-Time Integrator/3, Sum/1
  Product/1 -> Sum1/2

== system mach_lib/claw_main/att_loops/select att cmd ==
  e_current : Inport
  throt_current : Inport  Port=2
  outer cmd : Inport  Port=3
  signal_bus : Inport  Port=4
  Bus Selector1 : BusSelector  OutputSignals=cmd_bus.select_cmd.att
  Compare To Zero : simulink/Logic and Bit Operations/Compare To Zero  relop===  LogicOutDataTypeMode=boolean  ZeroCross=off
  Demux : Demux  Outputs=[ 4 1 ]
  Demux1 : Demux  Outputs=[ 3 MACH.num_u_throt ]
  Demux2 : Demux  Outputs=[ 1 3 ]
  Mux1 : Mux  Inputs=2
  Switch : Switch  Threshold=0.5
  Unit Delay2 : UnitDelay  X0=MACH_throttle_IC  SampleTime=-1
  att2e_ref : utility_lib/att2e_ref
  e2att : utility_lib/e2att
  get direct cmd : Subsystem
  switch att cmd : MultiPortSwitch  Inputs=3  zeroidx=on  SaturateOnIntegerOverflow=on
  switch throt cmd : MultiPortSwitch  Inputs=3  zeroidx=on  SaturateOnIntegerOverflow=on
  e_cmd : Outport
  throt_cmd : Outport  Port=2
  cmd : Outport  Port=3
  wires:
  Mux1/1 -> cmd/1
  Compare To Zero/1 -> Switch/2
  Demux2/2 -> switch att cmd/1
  Demux2/1 -> Compare To Zero/1
  Switch/1 -> e_cmd/1
  att2e_ref/1 -> Switch/3
  Demux1/1 -> switch att cmd/4
  e2att/1 -> switch att cmd/2
  get direct cmd/1(att) -> switch att cmd/3
  Unit Delay2/1 -> switch throt cmd/2
  e_current/1 -> att2e_ref/2, Switch/1, e2att/1
  Demux/1 -> Demux2/1
  signal_bus/1 -> Bus Selector1/1, get direct cmd/1(signal_bus)
  switch throt cmd/1 -> Mux1/2, throt_cmd/1
  Demux1/2 -> switch throt cmd/4
  outer cmd/1 -> Demux1/1
  Demux/2 -> switch throt cmd/1
  throt_current/1 -> Unit Delay2/1
  get direct cmd/2(throt) -> switch throt cmd/3
  Bus Selector1/1 -> Demux/1  "<att>"
  switch att cmd/1 -> Mux1/1, att2e_ref/1

== system mach_lib/claw_main/grab ExportedGlobal/grab cv variables ==
  In1 : Inport
  Bus Selector6 : BusSelector  OutputSignals=rate.cv,att.cv,vel.cv,pos.cv
  Demux1 : Demux  Outputs=3
  Demux2 : Demux
  Demux3 : Demux  Outputs=3
  Demux4 : Demux  Outputs=3
  Mux : Mux  Inputs=13
  Subsystem : Subsystem  TreatAsAtomicUnit=on
      settings: RTWSystemCode=Inline
  Out1 : Outport
  wires:
  Bus Selector6/4 -> Demux4/1  "<cv>"
  Bus Selector6/3 -> Demux3/1  "<cv>"
  Bus Selector6/2 -> Demux2/1  "<cv>"
  Bus Selector6/1 -> Demux1/1  "<cv>"
  Demux4/3 -> Subsystem/13(In13)
  Demux4/2 -> Subsystem/12(In12)
  Demux4/1 -> Subsystem/11(In11)
  Demux3/3 -> Subsystem/10(In10)
  Demux3/2 -> Subsystem/9(In9)
  Demux3/1 -> Subsystem/8(In8)
  Demux2/4 -> Subsystem/7(In7)
  Demux2/3 -> Subsystem/6(In6)
  Demux2/2 -> Subsystem/5(In5)
  Demux2/1 -> Subsystem/4(In4)
  Demux1/3 -> Subsystem/3(In3)
  Demux1/2 -> Subsystem/2(In2)
  Demux1/1 -> Subsystem/1(In1)
  Mux/1 -> Out1/1
  In1/1 -> Bus Selector6/1
  Subsystem/7(Out7) -> Mux/7  "CLAW_e3_cv"
  Subsystem/13(Out13) -> Mux/13  "CLAW_h_cv"
  Subsystem/12(Out12) -> Mux/12  "CLAW_E_cv"
  Subsystem/11(Out11) -> Mux/11  "CLAW_N_cv"
  Subsystem/10(Out10) -> Mux/10  "CLAW_hdot_cv"
  Subsystem/9(Out9) -> Mux/9  "CLAW_Edot_cv"
  Subsystem/8(Out8) -> Mux/8  "CLAW_Ndot_cv"
  Subsystem/6(Out6) -> Mux/6  "CLAW_e2_cv"
  Subsystem/5(Out5) -> Mux/5  "CLAW_e1_cv"
  Subsystem/4(Out4) -> Mux/4  "CLAW_e0_cv"
  Subsystem/3(Out3) -> Mux/3  "CLAW_r_cv"
  Subsystem/2(Out2) -> Mux/2  "CLAW_q_cv"
  Subsystem/1(Out1) -> Mux/1  "CLAW_p_cv"

== system mach_lib/claw_main/grab ExportedGlobal/grab cvcmd variables ==
  In1 : Inport
  Bus Selector5 : BusSelector  OutputSignals=rate.cvc,att.cvc,vel.cvc,pos.cvc
  Demux1 : Demux  Outputs=3
  Demux2 : Demux
  Demux3 : Demux  Outputs=3
  Demux4 : Demux  Outputs=3
  Mux : Mux  Inputs=13
  Subsystem : Subsystem  TreatAsAtomicUnit=on
      settings: RTWSystemCode=Inline
  Out1 : Outport
  wires:
  Bus Selector5/3 -> Demux3/1  "<cvc>"
  Bus Selector5/1 -> Demux1/1  "<cvc>"
  Bus Selector5/2 -> Demux2/1  "<cvc>"
  Bus Selector5/4 -> Demux4/1  "<cvc>"
  Demux4/3 -> Subsystem/13(In13)
  Demux4/2 -> Subsystem/12(In12)
  Demux4/1 -> Subsystem/11(In11)
  Demux3/3 -> Subsystem/10(In10)
  Demux3/2 -> Subsystem/9(In9)
  Demux3/1 -> Subsystem/8(In8)
  Demux2/4 -> Subsystem/7(In7)
  Demux2/3 -> Subsystem/6(In6)
  Demux2/2 -> Subsystem/5(In5)
  Demux2/1 -> Subsystem/4(In4)
  Demux1/3 -> Subsystem/3(In3)
  Demux1/2 -> Subsystem/2(In2)
  Demux1/1 -> Subsystem/1(In1)
  Mux/1 -> Out1/1
  In1/1 -> Bus Selector5/1
  Subsystem/7(Out7) -> Mux/7  "CLAW_e3_cvcmd"
  Subsystem/13(Out13) -> Mux/13  "CLAW_h_cvcmd"
  Subsystem/12(Out12) -> Mux/12  "CLAW_E_cvcmd"
  Subsystem/11(Out11) -> Mux/11  "CLAW_N_cvcmd"
  Subsystem/10(Out10) -> Mux/10  "CLAW_hdot_cvcmd"
  Subsystem/9(Out9) -> Mux/9  "CLAW_Edot_cvcmd"
  Subsystem/8(Out8) -> Mux/8  "CLAW_Ndot_cvcmd"
  Subsystem/6(Out6) -> Mux/6  "CLAW_e2_cvcmd"
  Subsystem/5(Out5) -> Mux/5  "CLAW_e1_cvcmd"
  Subsystem/4(Out4) -> Mux/4  "CLAW_e0_cvcmd"
  Subsystem/3(Out3) -> Mux/3  "CLAW_r_cvcmd"
  Subsystem/2(Out2) -> Mux/2  "CLAW_q_cvcmd"
  Subsystem/1(Out1) -> Mux/1  "CLAW_p_cvcmd"

== system mach_lib/claw_main/grab ExportedGlobal/grab cvdex variables ==
  In1 : Inport
  Bus Selector3 : BusSelector  OutputSignals=rate.cvdex,att.cvdex,vel.cvdex,pos.cvdex
  Demux1 : Demux  Outputs=3
  Demux2 : Demux
  Demux3 : Demux  Outputs=3
  Demux4 : Demux  Outputs=3
  Mux : Mux  Inputs=13
  Subsystem : Subsystem  TreatAsAtomicUnit=on
      settings: RTWSystemCode=Inline
  Out1 : Outport
  wires:
  Bus Selector3/1 -> Demux1/1  "<cvdex>"
  Bus Selector3/2 -> Demux2/1  "<cvdex>"
  Bus Selector3/3 -> Demux3/1  "<cvdex>"
  Bus Selector3/4 -> Demux4/1  "<cvdex>"
  In1/1 -> Bus Selector3/1
  Mux/1 -> Out1/1
  Demux4/3 -> Subsystem/13(In13)
  Demux4/2 -> Subsystem/12(In12)
  Demux4/1 -> Subsystem/11(In11)
  Demux3/3 -> Subsystem/10(In10)
  Demux3/2 -> Subsystem/9(In9)
  Demux3/1 -> Subsystem/8(In8)
  Demux2/4 -> Subsystem/7(In7)
  Demux2/3 -> Subsystem/6(In6)
  Demux2/2 -> Subsystem/5(In5)
  Demux2/1 -> Subsystem/4(In4)
  Demux1/3 -> Subsystem/3(In3)
  Demux1/2 -> Subsystem/2(In2)
  Demux1/1 -> Subsystem/1(In1)
  Subsystem/7(Out7) -> Mux/7  "CLAW_e3_cvdex"
  Subsystem/13(Out13) -> Mux/13  "CLAW_h_cvdex"
  Subsystem/12(Out12) -> Mux/12  "CLAW_E_cvdex"
  Subsystem/11(Out11) -> Mux/11  "CLAW_N_cvdex"
  Subsystem/10(Out10) -> Mux/10  "CLAW_hdot_cvdex"
  Subsystem/9(Out9) -> Mux/9  "CLAW_Edot_cvdex"
  Subsystem/8(Out8) -> Mux/8  "CLAW_Ndot_cvdex"
  Subsystem/6(Out6) -> Mux/6  "CLAW_e2_cvdex"
  Subsystem/5(Out5) -> Mux/5  "CLAW_e1_cvdex"
  Subsystem/4(Out4) -> Mux/4  "CLAW_e0_cvdex"
  Subsystem/3(Out3) -> Mux/3  "CLAW_r_cvdex"
  Subsystem/2(Out2) -> Mux/2  "CLAW_q_cvdex"
  Subsystem/1(Out1) -> Mux/1  "CLAW_p_cvdex"

== system mach_lib/claw_main/grab ExportedGlobal/grab integrator variables ==
  In1 : Inport
  Bus Selector4 : BusSelector  OutputSignals=rate.integ,att.integ,vel.integ,pos.integ
  Demux1 : Demux  Outputs=3
  Demux2 : Demux
  Demux3 : Demux  Outputs=3
  Demux4 : Demux  Outputs=3
  Mux : Mux  Inputs=13
  Subsystem : Subsystem  TreatAsAtomicUnit=on
      settings: RTWSystemCode=Inline
  Out1 : Outport
  wires:
  Bus Selector4/1 -> Demux1/1  "<integ>"
  Bus Selector4/2 -> Demux2/1  "<integ>"
  Bus Selector4/3 -> Demux3/1  "<integ>"
  Bus Selector4/4 -> Demux4/1  "<integ>"
  In1/1 -> Bus Selector4/1
  Demux4/3 -> Subsystem/13(In13)
  Demux4/2 -> Subsystem/12(In12)
  Demux4/1 -> Subsystem/11(In11)
  Demux3/3 -> Subsystem/10(In10)
  Demux3/2 -> Subsystem/9(In9)
  Demux3/1 -> Subsystem/8(In8)
  Demux2/4 -> Subsystem/7(In7)
  Demux2/3 -> Subsystem/6(In6)
  Demux2/2 -> Subsystem/5(In5)
  Demux2/1 -> Subsystem/4(In4)
  Demux1/3 -> Subsystem/3(In3)
  Demux1/2 -> Subsystem/2(In2)
  Demux1/1 -> Subsystem/1(In1)
  Mux/1 -> Out1/1
  Subsystem/7(Out7) -> Mux/7  "CLAW_e3_int"
  Subsystem/13(Out13) -> Mux/13  "CLAW_h_int"
  Subsystem/12(Out12) -> Mux/12  "CLAW_E_int"
  Subsystem/11(Out11) -> Mux/11  "CLAW_N_int"
  Subsystem/10(Out10) -> Mux/10  "CLAW_hdot_int"
  Subsystem/9(Out9) -> Mux/9  "CLAW_Edot_int"
  Subsystem/8(Out8) -> Mux/8  "CLAW_Ndot_int"
  Subsystem/6(Out6) -> Mux/6  "CLAW_e2_int"
  Subsystem/5(Out5) -> Mux/5  "CLAW_e1_int"
  Subsystem/4(Out4) -> Mux/4  "CLAW_e0_int"
  Subsystem/3(Out3) -> Mux/3  "CLAW_r_int"
  Subsystem/2(Out2) -> Mux/2  "CLAW_q_int"
  Subsystem/1(Out1) -> Mux/1  "CLAW_p_int"

== system mach_lib/claw_main/grab ExportedGlobal/grab w_est variables ==
  In1 : Inport
  Bus Selector12 : BusSelector  OutputSignals=w_est_debug.w_est
  Demux1 : Demux  Outputs=3
  Mux : Mux  Inputs=3
  Subsystem : Subsystem  TreatAsAtomicUnit=on
      settings: RTWSystemCode=Inline
  Out1 : Outport
  wires:
  In1/1 -> Bus Selector12/1
  Bus Selector12/1 -> Demux1/1  "<w_est>"
  Mux/1 -> Out1/1
  Demux1/3 -> Subsystem/3(In3)
  Demux1/2 -> Subsystem/2(In2)
  Demux1/1 -> Subsystem/1(In1)
  Subsystem/3(Out3) -> Mux/3  "CLAW_Dd_wind"
  Subsystem/2(Out2) -> Mux/2  "CLAW_Ed_wind"
  Subsystem/1(Out1) -> Mux/1  "CLAW_Nd_wind"

== system mach_lib/claw_main/input processing/mode dependent stick processing ==
  command : Inport
  signal_bus : Inport  Port=2
  Bus Creator : BusCreator  Inputs=2
  Bus Selector1 : BusSelector  OutputSignals=control_params.accel_cmd_sw,mode_sw.CLAW_mode
  Bus Selector2 : BusSelector  OutputSignals=y_meas.NEh_dot,x_est
  att rate cmd : Subsystem
  att_type cmd : Subsystem
  feed forward : Subsystem
  llh cmd : Subsystem
  rampin vel_cmd : Subsystem
  set command selection switches : Subsystem
  table iv computation : Subsystem
  use table lookup pos cmds : Subsystem
  cmd_bus : Outport
  feed_forward : Outport  Port=2
  wires:
  att rate cmd/1(command_out) -> att_type cmd/2(command_in)
  att_type cmd/1(command_out) -> rampin vel_cmd/2(command_in)
  command/1 -> llh cmd/2(command_in)
  feed forward/1(feed_forward) -> feed_forward/1
  table iv computation/1(table_bus) -> feed forward/1(table_bus), use table lookup pos cmds/3(table_bus)
  Bus Selector2/2 -> table iv computation/1(x_est)  "<x_est>"
  use table lookup pos cmds/1(command_out) -> Bus Creator/2  "autopilot_cmd"
  Bus Creator/1 -> cmd_bus/1
  rampin vel_cmd/1(command_out) -> use table lookup pos cmds/2(command_in)
  set command selection switches/1(select_cmd) -> Bus Creator/1  "select_cmd"
  Bus Selector1/1 -> set command selection switches/1(accel_cmd_sw)  "<accel_cmd_sw>"
  Bus Selector2/1 -> rampin vel_cmd/3(NEh_dot)  "<NEh_dot>"
  llh cmd/1(command_out) -> att rate cmd/2(command_in)
  signal_bus/1 -> feed forward/2(signal_bus), att_type cmd/3(signal_bus), Bus Selector2/1, att rate cmd/3(signal_bus), llh cmd/3(signal_bus), Bus Selector1/1
  Bus Selector1/2 -> att_type cmd/1(mode), use table lookup pos cmds/1(mode), rampin vel_cmd/1(mode), llh cmd/1(mode), att rate cmd/1(mode), set command selection switches/2(CLAW_mode)  "<CLAW_mode>"

== system mach_lib/claw_main/input processing/modify limits and apply to direct commands ==
  note: Currently, the limits for direct mode and throttle in att and rate modes
      | are the same as those used for automatic control.  May want to revisit this someday ...
  u_old : Inport
  u_meas : Inport  Port=2
  full_surf_in : Inport  Port=3
  Bus Assignment : BusAssignment  AssignedSignals=full_surf_cmd
  Bus Selector2 : BusSelector  OutputSignals=full_surf_ulim,full_surf_llim,full_surf_urlim,full_surf_lrlim,full_surf_cmd
  MinMax : MinMax  Inputs=2  SaturateOnIntegerOverflow=on  InputSameDT=on
  MinMax2 : MinMax  Function=max  Inputs=2  SaturateOnIntegerOverflow=on  InputSameDT=on
  apply surface locking : Subsystem
  limit computation : mach_lib/limit computation
  rate limit limits : mach_lib/rate limit limits  ulim=MACH.u_ulim  llim=MACH.u_llim
  throt out of fuel limits : Subsystem
  full_surf : Outport
  wires:
  apply surface locking/1(full_surf) -> throt out of fuel limits/1(full_surf_in)
  full_surf_in/1 -> apply surface locking/2(full_surf_in)
  u_meas/1 -> apply surface locking/1(u_meas)
  Bus Assignment/1 -> full_surf/1
  Bus Selector2/1 -> rate limit limits/2  "<full_surf_ulim>"
  throt out of fuel limits/1(full_surf) -> Bus Assignment/1, Bus Selector2/1
  MinMax/1 -> Bus Assignment/2
  Bus Selector2/5 -> MinMax2/2  "<full_surf_cmd>"
  Bus Selector2/2 -> rate limit limits/3  "<full_surf_llim>"
  u_old/1 -> limit computation/1, rate limit limits/1
  MinMax2/1 -> MinMax/2
  limit computation/1 -> MinMax/1
  limit computation/2 -> MinMax2/1
  rate limit limits/2 -> limit computation/3
  rate limit limits/1 -> limit computation/2
  Bus Selector2/4 -> limit computation/5, rate limit limits/5  "<full_surf_lrlim>"
  Bus Selector2/3 -> limit computation/4, rate limit limits/4  "<full_surf_urlim>"

== system mach_lib/claw_main/input processing/select att_type ==
  scoped_bus : Inport
  mode_sw_in : Inport  Port=2
  signal_bus : Inport  Port=3
  Bus Assignment : BusAssignment  AssignedSignals=att_type
  Bus Selector : BusSelector  OutputSignals=qbar,abs_vel_rw,abs_cos_beta,abs_cos_theta,abs_cos_b,abs_cos_gamma_rw
  Bus Selector1 : BusSelector  OutputSignals=att_type
  Constant5 : Constant  Value=use_auto_att_type
  Multiport Switch1 : MultiPortSwitch  Inputs=2  zeroidx=on
  Product : Product  RndMeth=Zero
  add tiebreaker for current att_type : Subsystem
  att type input : Scope  NumInputPorts=6
      settings: YMin=1~0~0~0.1~5.55112e-017~5.55112e-017  YMax=4~900~5000~1~1~1  SaveName=att_type_input
  att type output : Scope  NumInputPorts=2
      settings: YMin=1~0  YMax=4~2.5  SaveName=att_type_output
  compute precond vars : Subsystem
  evaluate preconditions : Subsystem
  priority_weighting : Constant  Value=[0 1 1 0 2 0]
  select best att_type : Subsystem
  mode_sw : Outport
  wires:
  Bus Selector/6 -> att type input/6  "<abs_cos_gamma_rw>"
  Bus Selector/5 -> att type input/5  "<abs_cos_b>"
  Bus Selector/4 -> att type input/4  "<abs_cos_theta>"
  Bus Selector/3 -> att type input/3  "<abs_cos_beta>"
  Bus Selector/2 -> att type input/2  "<abs_vel_rw>"
  Bus Selector/1 -> att type input/1  "<qbar>"
  compute precond vars/1(precond_vars) -> evaluate preconditions/1(precond_vars), Bus Selector/1
  priority_weighting/1 -> add tiebreaker for current att_type/2(priority_in)
  Constant5/1 -> Multiport Switch1/1
  Multiport Switch1/1 -> Bus Assignment/2
  evaluate preconditions/1(precond_satisfied) -> Product/2
  select best att_type/1(idx_max) -> add tiebreaker for current att_type/1(att_type_selected), Multiport Switch1/3, att type output/1  "att_type_selected"
  Product/1 -> att type output/2, select best att_type/1(vec)  "att_type_availability"
  add tiebreaker for current att_type/1(priority_out) -> Product/1
  Bus Assignment/1 -> mode_sw/1
  Bus Selector1/1 -> Multiport Switch1/2  "<att_type>"
  signal_bus/1 -> compute precond vars/1(signal_bus)
  mode_sw_in/1 -> Bus Assignment/1, Bus Selector1/1
  scoped_bus/1 -> compute precond vars/2(scoped_bus)
